simulink model "IEEE34bus_v2019b_Phasor_DPL_ZIPload"  (R2019b)
(part 2 of 9)

  846-848 301/LConn2 -- 846 Y PQ1/LConn1 -- 846/RConn2
  834 D Z/LConn2 -- 834/RConn2 -- 834-860 301/LConn2 -- 834-842 301/LConn2
  834-860 301/RConn3 -- 860 Y PQ/LConn3 -- 860/LConn3 -- 860 D Z/LConn3
  830-854 301/RConn1 -- 854/LConn1
  834-860 301/LConn1 -- 834-842 301/LConn1 -- 834 D Z/LConn1 -- 834/RConn1
  842/RConn3 -- 842-844 301/LConn3
  830-854 301/RConn2 -- 854/LConn2
  846/RConn1 -- 846-848 301/LConn1
  832-858 301/RConn1 -- 858/LConn1
  844-846 301/LConn3 -- 844 Y Z/LConn3 -- 844/RConn3 -- 844 Yg Z/LConn3 -- 844 Y PQ1/LConn3
  842/RConn2 -- 842-844 301/LConn2
  844-846 301/LConn1 -- 844 Y Z/LConn1 -- 844/RConn1 -- 844 Yg Z/LConn1 -- 844 Y PQ1/LConn1
  832-858 301/RConn2 -- 858/LConn2
  830-854 301/RConn3 -- 854/LConn3
  842-844 301/LConn1 -- 842 Y PQ/LConn1 -- 842/RConn1
  834-860 301/RConn1 -- 860 Y PQ/LConn1 -- 860/LConn1 -- 860 D Z/LConn1
  830/RConn1 -- 830 D Z/LConn1 -- 830-854 301/LConn1
  830/RConn2 -- 830 D Z/LConn2 -- 830-854 301/LConn2
  844-846 301/RConn3 -- 846 Y PQ/LConn3 -- 846/LConn3
  844-846 301/RConn2 -- 846 Y PQ/LConn2 -- 846/LConn2
  832-858 301/RConn3 -- 858/LConn3
  844-846 301/LConn2 -- 844 Y Z/LConn2 -- 844/RConn2 -- 844 Yg Z/LConn2 -- 844 Y PQ1/LConn2
  830/RConn3 -- 830 D Z/LConn3 -- 830-854 301/LConn3
  834-860 301/RConn2 -- 860 Y PQ/LConn2 -- 860/LConn2 -- 860 D Z/LConn2
  844-846 301/RConn1 -- 846 Y PQ/LConn1 -- 846/LConn1
  818-820 302/LConn1 -- 818 Y Z/LConn1 -- 818/LConn1
  808-812 300/LConn3 -- 808/RConn3
  816-824 301/LConn3 -- 816 D I/LConn3 -- "816 "/RConn3
  806-808 300/RConn3 -- 808/LConn3
  "816 "/RConn1 -- 816 D I/LConn1 -- 816-824 301/LConn1 -- 816-818 302/LConn1
  816-824 301/RConn3 -- 824 D I/LConn3 -- 824 Y PQ/LConn1 -- 824-828 301/LConn3 -- "824 "/LConn3
  808-812 300/LConn1 -- 808/RConn1
  806-808 300/RConn2 -- 808/LConn2
  824-826 303/LConn1 -- 824 Y I/LConn1 -- "824 "/RConn2
  828/RConn2 -- 828-830 301/LConn2
  830/LConn2 -- 828-830 301/RConn2
  808-810 303/LConn1 -- 808 Y I/LConn1 -- 808-812 300/LConn2 -- 808/RConn2
  820/LConn1 -- 820 Y PQ/LConn1 -- 820-822 302/LConn1
  828/RConn3 -- 828-830 301/LConn3
  "816 "/RConn2 -- 816 D I/LConn2 -- 816-824 301/LConn2
  828-830 301/LConn1 -- 828 Y PQ1/LConn1 -- 828/RConn1
  828/LConn2 -- 824-828 301/RConn2
  830/LConn3 -- 828-830 301/RConn3
  828/LConn1 -- 824-828 301/RConn1
  824 D I/LConn2 -- 816-824 301/RConn2 -- 824-828 301/LConn2 -- "824 "/LConn2
  828-830 301/RConn1 -- 830 Y PQ/LConn1 -- 830/LConn1
  824-828 301/RConn3 -- 828/LConn3 -- 828 Y PQ/LConn1
  816-824 301/RConn1 -- 824 D I/LConn1 -- 824-828 301/LConn1 -- "824 "/LConn1
  802-806 300/RConn1 -- 806/LConn1
  802-806 300/LConn3 -- 802/RConn3 -- 802 Y PQ/LConn3
  800-802 300/RConn2 -- 802/LConn2
  806-808 300/LConn2 -- 806 Y PQ/LConn2 -- 806/RConn2
  806-808 300/LConn1 -- 806 Y PQ/LConn1 -- 806/RConn1
  802-806 300/RConn3 -- 806/LConn3
  802-806 300/LConn1 -- 802/RConn1 -- 802 Y PQ/LConn1
  806-808 300/RConn1 -- 808/LConn1
  800-802 300/RConn3 -- 802/LConn3
  802-806 300/LConn2 -- 802/RConn2 -- 802 Y PQ/LConn2
  806-808 300/LConn3 -- 806 Y PQ/LConn3 -- 806/RConn3
  802-806 300/RConn2 -- 806/LConn2
  800-802 300/RConn1 -- 802/LConn1
  Regulator 1/LConn1 -- 814/RConn1
  Regulator 1/LConn2 -- 814/RConn2
  Regulator 1/LConn3 -- 814/RConn3
  Regulator 1/RConn1 -- RG10/LConn1
  Regulator 1/RConn2 -- RG10/LConn2
  Regulator 1/RConn3 -- RG10/LConn3
  Regulator 2/LConn1 -- "852 "/RConn1
  Regulator 2/LConn2 -- "852 "/RConn2
  Regulator 2/LConn3 -- "852 "/RConn3
  Regulator 2/RConn1 -- RG11/LConn1
  Regulator 2/RConn2 -- RG11/LConn2
  Regulator 2/RConn3 -- RG11/LConn3
  Ground15/LConn1 -- 824 Y PQ/RConn1
  Ground18/LConn1 -- 830 Y PQ/RConn1
  Ground19/LConn1 -- 844 Y PQ/RConn1
  Ground20/LConn1 -- 842 Y PQ/RConn1
  Ground21/LConn1 -- 848 Y PQ/RConn1
  Ground22/LConn1 -- 846 Y PQ1/RConn1
  Ground16/LConn1 -- 828 Y PQ/RConn1
  Ground17/LConn1 -- 828 Y PQ1/RConn1
  800-802 300/LConn3 -- 800/RConn3
  800-802 300/LConn2 -- 800/RConn2
  800-802 300/LConn1 -- 800/RConn1
  854-852 301/RConn1 -- "852 "/LConn1
  854-852 301/RConn2 -- "852 "/LConn2
  854-852 301/RConn3 -- "852 "/LConn3
  834-842 301/RConn1 -- 842/LConn1
  834-842 301/RConn2 -- 842/LConn2
  834-842 301/RConn3 -- 842/LConn3
